simulink model "Lab1_parameter_estimation_student"  (R2024b)
settings: Solver=FixedStepAuto  StartTime=0.0  StopTime=10  FixedStep=0.001  RelTol=1e-3
values from neighbouring files (symbols this model uses):
  motor_B = 0.0001    [Lab1_motor_params_student.m]
  motor_Eff = 0.5    [Lab1_motor_params_student.m]
  motor_J = 0.001    [Lab1_motor_params_student.m]
  motor_Ke = 0.05    [Lab1_motor_params_student.m]
  motor_L = 0.0038    [Lab1_motor_params_student.m]
  motor_R = 5.54    [Lab1_motor_params_student.m]
libraries: simulink x1
settings Model: Creator=tanawatp  LastModifiedBy=acer
settings RTWCC: GPUComputeCapability=3.5

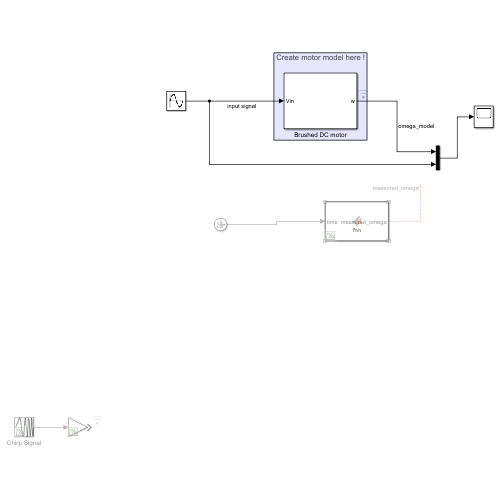
[thumbnail: Simulink's stored preview of the top-level diagram]
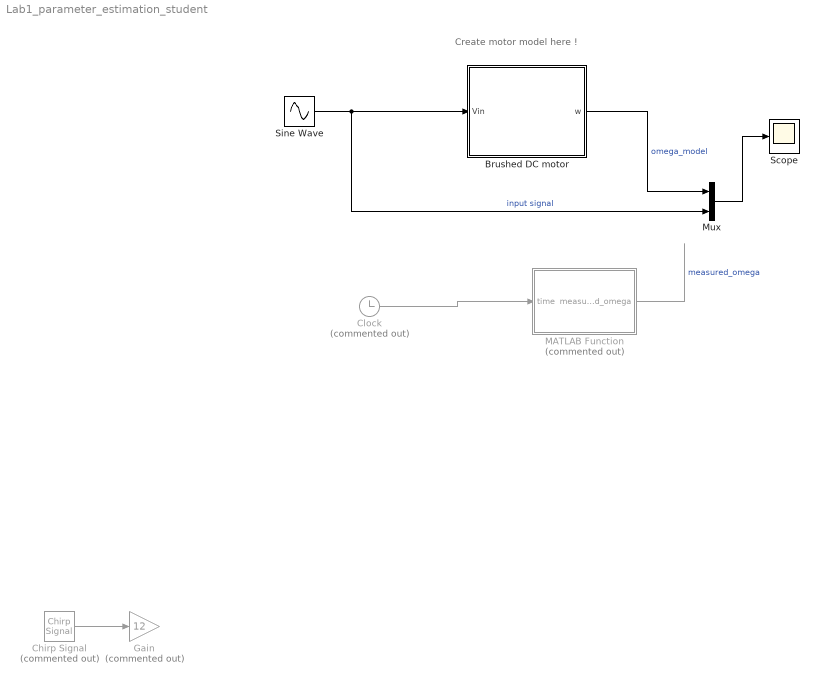
== system Lab1_parameter_estimation_student ==
  note: Create motor model here !
  Brushed DC motor : Subsystem
  Chirp Signal : simulink/Sources/Chirp Signal  Commented=on  f1=0.1  T=40  f2=5
  Clock : Clock  Commented=on
  Gain : Gain  Commented=on  Gain=12
  MATLAB Function : MATLAB Function  Commented=on  TreatAsAtomicUnit=on
  Mux : Mux  Inputs=2
  Scope : Scope
  Sine Wave : Sin  Amplitude=12  Frequency=2*pi*0.1  SampleTime=0
  wires:
  Brushed DC motor/1(w) -> Mux/1  "omega_model"
  Chirp Signal/1 -> Gain/1
  Sine Wave/1 -> Mux/2, Brushed DC motor/1(Vin)  "input signal"
  Mux/1 -> Scope/1
  Clock/1 -> MATLAB Function/1(time)
  MATLAB Function/1(measured_omega) -> ?  "measured_omega"

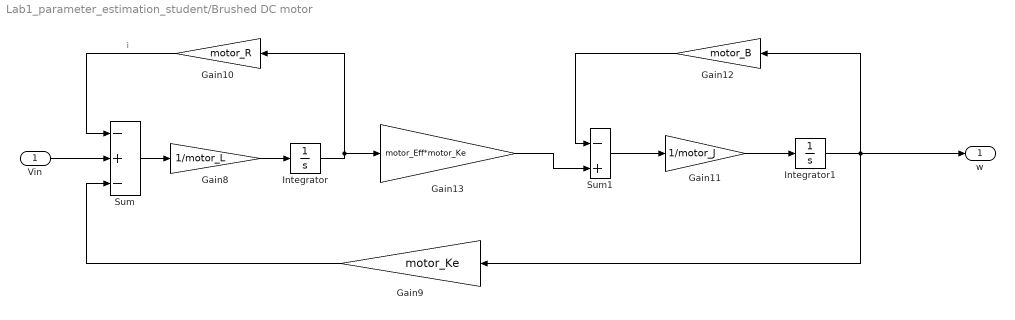
== system Lab1_parameter_estimation_student/Brushed DC motor ==
  Vin : Inport
  Gain10 : Gain  Gain=motor_R
  Gain11 : Gain  Gain=1/motor_J
  Gain12 : Gain  Gain=motor_B
  Gain13 : Gain  Gain=motor_Eff*motor_Ke
  Gain8 : Gain  Gain=1/motor_L
  Gain9 : Gain  Gain=motor_Ke
  Integrator : Integrator
  Integrator1 : Integrator
  Sum : Sum  Inputs=-+-
  Sum1 : Sum  Inputs=-|+|
  w : Outport
  wires:
  Vin/1 -> Sum/2
  Sum/1 -> Gain8/1
  Gain8/1 -> Integrator/1
  Integrator/1 -> Gain10/1, Gain13/1
  Gain10/1 -> Sum/1  "i"
  Gain13/1 -> Sum1/2
  Sum1/1 -> Gain11/1
  Integrator1/1 -> Gain9/1, Gain12/1, w/1
  Gain12/1 -> Sum1/1
  Gain11/1 -> Integrator1/1
  Gain9/1 -> Sum/3

== matlab function Lab1_parameter_estimation_student/MATLAB Function ==
  data: time input; measured_omega output
function measured_omega = fcn(time)
    global Time Velo;
    idx = find(abs(Time - time) <= 1e-6, 1);
    measured_omega = Velo(idx);
    %{
    if ~isempty(idx)
        measured_omega = Velo(idx);
    else
        measured_omega = -1;
    end

    measured_omega = Velo(1);
    %}
end
